simulink model "parking"  (R2025b)
settings: Solver=ode5  StartTime=0.0  StopTime=15  FixedStep=1e-3  RelTol=1e-3
libraries: dspsigops x2
settings Model: Creator=Cris  LastModifiedBy=Cris

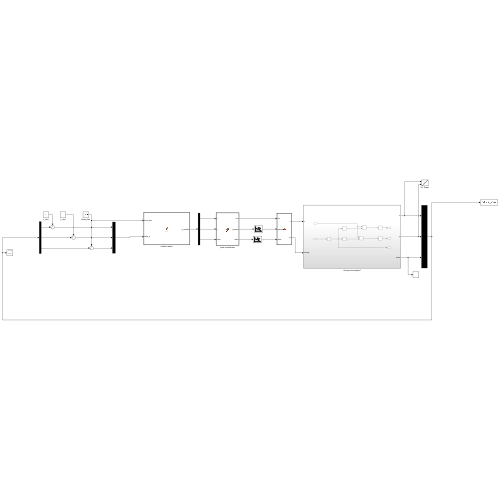
[thumbnail: Simulink's stored preview of the top-level diagram]
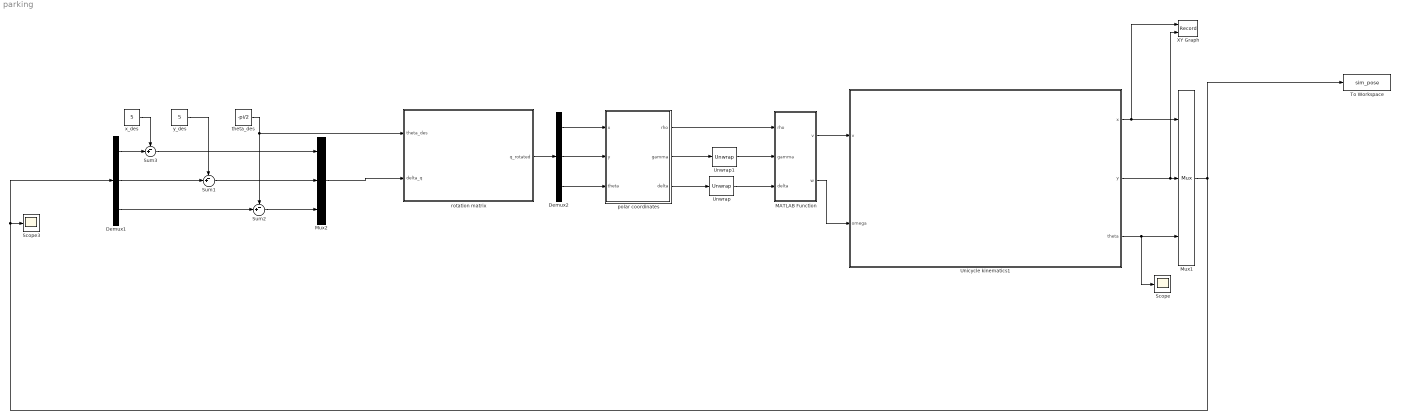
== system parking ==
  Demux1 : Demux  Outputs=3
  Demux2 : Demux  Outputs=3
  MATLAB Function : MATLAB Function  TreatAsAtomicUnit=on
  Mux1 : Mux  Inputs=3
  Mux2 : Mux  Inputs=3
  Scope : Scope
      settings: ActiveDisplayYMinimum=-1  ActiveDisplayYMaximum=1
  Scope3 : Scope
      settings: ActiveDisplayYMinimum=-1  ActiveDisplayYMaximum=1  DataLoggingVariableName=ScopeData4
  Sum1 : Sum  Inputs=-+|
  Sum2 : Sum  Inputs=-+|
  Sum3 : Sum  Inputs=-+|
  To Workspace : ToWorkspace  VariableName=sim_pose  SaveFormat=Timeseries  SampleTime=-1
  Unicycle kinematics1 : Subsystem
  Unwrap : dspsigops/Unwrap  tol=pi  InputProcessing=Columns as channels (frame based)  running=off
  Unwrap1 : dspsigops/Unwrap  tol=pi  InputProcessing=Columns as channels (frame based)  running=off
  XY Graph : Record  NumPorts=2.0  FileSettingsInternal="{\"entries\":[{\"content\":{\"excelSettings\":{\"content\":{},\"type\":\"Streamout.ExcelSettings\"},\"parquetSettings\":{\"content\":{},\"type\":\"Streamout.ParquetSettings\"}},\"type\":\"Streamout.FileSettingStorage\",\"uuid\":\"\"}],\"packageUris\":[\"http:\\/\\/schema.mathworks.com\\/mf0\\/streamout_blocks\\/R2020a\"],\"version\":\"1.0\"}"  FrameSettings=[0, 0]  Layout=[1 1]  SignalsInternal="{\"entries\":[{\"content\":{\"signals\":[{\"content\":{\"blockPath\":[],\"dimensions\":[1],\"domain\":\"\",\"lineColor\":\"#a2142f\",\"plots\":[ 1 ],\"port\":1,\"sid\":[\"\"],\"signalID\":1,\"signalName\":\"Unicycle kinematics1:1\"},\"type\":\"RecordBlkView.Signal\",\"uuid\":\"\"},{\"content\":{\"blockPath\":[],\"dimensions\":[1],\"domain\":\"\",\"lineColor\":\"#139fff\",\"plots\":[ 1 ],\"port\":2,\"sid\":[\"\"],\"signalID\":2,\"signalName\":\"Unicycle kinematics1:2\"},\"type\":\"RecordBlkView.Signal\",\"uuid\":\"\"}]},\"type\":\"RecordBlkView.InputSignals\",\"uuid\":\"\"}],\"packageUris\":[\"http:\\/\\/schema.mathworks.com\\/mf0\\/streamout_blocks\\/R2020a\"],\"version\":\"1.0\"}"  VisualizationBindings="{\"xyplotplugin\":{\"info\":[{\"series\":[{\"bindingParametersList\":[{\"parameter\":\"X-Axis\",\"signalID\":1,\"signalName\":\"Unicycle kinematics1:1\"},{\"parameter\":\"Y-Axis\",\"signalID\":2,\"signalName\":\"Unicycle kinematics1:2\"}],\"seriesID\":0}],\"subplotID\":1}]}}"  CompatibilityTag=XY
  polar coordinates : MATLAB Function  TreatAsAtomicUnit=on
  rotation matrix : MATLAB Function  TreatAsAtomicUnit=on
  theta_des : Constant  Value=-pi/2
  x_des : Constant  Value=5
  y_des : Constant  Value=5
  wires:
  Unicycle kinematics1/2(y) -> XY Graph/2, Mux1/2
  MATLAB Function/2(w) -> Unicycle kinematics1/2(omega)
  Unicycle kinematics1/1(x) -> XY Graph/1, Mux1/1
  polar coordinates/1(rho) -> MATLAB Function/1(rho)
  Demux2/1 -> polar coordinates/1(x)
  Demux2/2 -> polar coordinates/2(y)
  rotation matrix/1(q_rotated) -> Demux2/1
  MATLAB Function/1(v) -> Unicycle kinematics1/1(v)
  Unicycle kinematics1/3(theta) -> Scope/1, Mux1/3
  y_des/1 -> Sum1/1
  Demux1/1 -> Sum3/2
  Demux1/2 -> Sum1/2
  Sum3/1 -> Mux2/1
  x_des/1 -> Sum3/1
  Demux1/3 -> Sum2/2
  Sum2/1 -> Mux2/3
  Mux1/1 -> To Workspace/1, Demux1/1, Scope3/1
  Mux2/1 -> rotation matrix/2(delta_q)
  Demux2/3 -> polar coordinates/3(theta)
  theta_des/1 -> Sum2/1, rotation matrix/1(theta_des)
  Sum1/1 -> Mux2/2
  polar coordinates/3(delta) -> Unwrap/1
  Unwrap/1 -> MATLAB Function/3(delta)
  polar coordinates/2(gamma) -> Unwrap1/1
  Unwrap1/1 -> MATLAB Function/2(gamma)

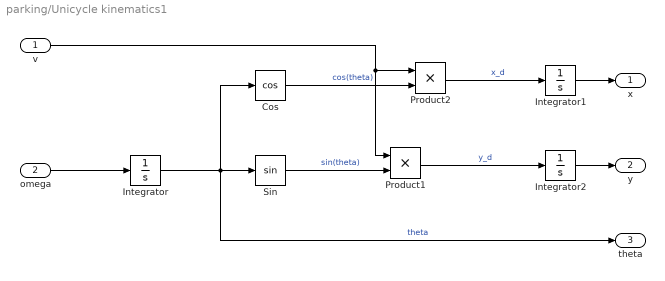
== system parking/Unicycle kinematics1 ==
  v : Inport
  omega : Inport  Port=2
  Cos : Trigonometry  Operator=cos
  Integrator : Integrator
  Integrator1 : Integrator
  Integrator2 : Integrator
  Product1 : Product
  Product2 : Product
  Sin : Trigonometry
  x : Outport
  y : Outport  Port=2
  theta : Outport  Port=3
  wires:
  omega/1 -> Integrator/1
  Integrator/1 -> theta/1, Cos/1, Sin/1  "theta"
  Cos/1 -> Product2/2  "cos(theta)"
  Sin/1 -> Product1/2  "sin(theta)"
  v/1 -> Product2/1, Product1/1
  Integrator1/1 -> x/1
  Product2/1 -> Integrator1/1  "x_d"
  Integrator2/1 -> y/1
  Product1/1 -> Integrator2/1  "y_d"

== matlab function parking/rotation matrix ==
  data: theta_des input; delta_q input; q_rotated output
function q_rotated  = fcn(theta_des, delta_q)

% rotation matrix
R = [cos(theta_des), sin(theta_des), 0;
    -sin(theta_des), cos(theta_des), 0; 
    0,              0,              1];

% rotate
q_rotated = R*delta_q;

== matlab function parking/MATLAB Function ==
  data: v output; rho input; gamma input; w output; delta input
function [v , w] = fcn(rho, gamma, delta)

% adjust gains
k1 = 5;%3
k2 = 5;%6
k3 = 5;%1.5


% controller

v = k1*rho*cos(gamma);

if (abs(gamma) > 0.001)
    temp = sin(gamma)/gamma;
else
    temp = 1;
end

w = k2*gamma + (k1*temp*cos(gamma))*(gamma+k3*delta);

if rho < 0.01
    v = 0;
    w = 0;
end

== matlab function parking/polar coordinates ==
  data: x input; rho output; gamma output; delta output; y input; theta input
function [rho, gamma, delta] = fcn(x, y, theta)

rho = sqrt(x^2+y^2);
gamma = atan2(y, x) + pi - theta;
delta = gamma + theta;
